simulink model "Speed_State_Feedback_PIL_Simulation"  (R2021b)
settings: Solver=VariableStepAuto  StartTime=0.0  StopTime=20  RelTol=1e-3  EnableMultiTasking=on
libraries: cstblocks x1
settings Model: SILPILSystemUnderTest=refmodels  ExtModeTrigDuration=10  Creator=UTENTE  LastModifiedBy=UTENTE
settings OptimizationCC: EnhancedBackFolding=on  PassReuseOutputArgsAs=Individual arguments  ZeroExternalMemoryAtStartup=off  ZeroInternalMemoryAtStartup=off  MaxStackSize=64  OptimizeBlockOrder=speed  DifferentSizesBufferReuse=on  OptimizationCustomize=off  EfficientTunableParamExpr=on
settings DebuggingCC: ParameterTunabilityLossMsg=error
settings HardwareCC: ProdBitPerPointer=32  ProdBitPerSizeT=32  ProdBitPerPtrDiffT=32  ProdLargestAtomicInteger=Long  ProdLargestAtomicFloat=Double  ProdWordSize=32  ProdLongLongMode=on  ProdHWDeviceType=ARM Compatible->ARM Cortex
settings SFSimCC: MATLABDynamicMemAlloc=off
settings RTWCC: Description=Embedded Coder  SystemTargetFile=ert.tlc  HardwareBoard=STM32 Nucleo F401RE  TemplateMakefile=ert_default_tmf  Toolchain=GNU Tools for ARM Embedded Processors  PortableWordSizes=on  CodeExecutionProfiling=on  CodeProfilingInstrumentation=coarse
settings CodeAppCC: ForceParamTrailComments=on  IgnoreCustomStorageClasses=off  OperatorAnnotations=on  SimulinkDataObjDesc=on  SFDataObjDesc=on  InsertBlockDesc=on
settings ERTTargetCC: ExtModeTransport=3  ExtModeStaticAlloc=on  ExtModeStaticAllocSize=2000  ExtModeMexFile=ext_xcp  ExtModeIntrfLevel=Level2 - Open

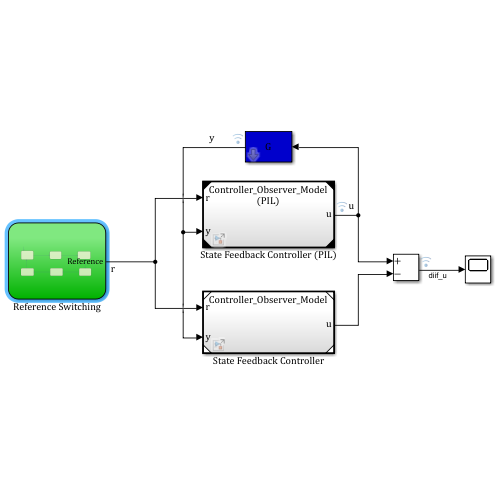
[thumbnail: Simulink's stored preview of the top-level diagram]
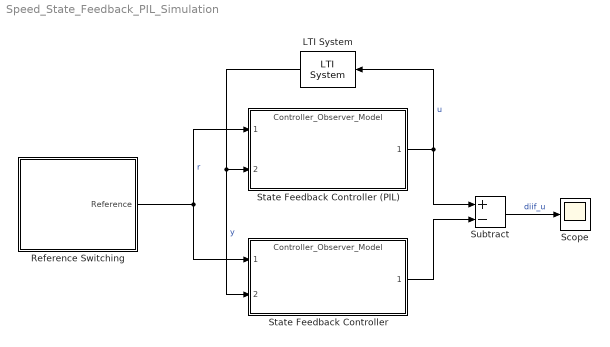
== system Speed_State_Feedback_PIL_Simulation ==
  LTI System : cstblocks/LTI System  sys=G  IC=[]
  Reference Switching : Stateflow chart  TreatAsAtomicUnit=on
  Scope : Scope
  State Feedback Controller : ModelReference  ModelNameDialog=Controller_Observer_Model.slx  SimulationMode=Normal  ModelReferenceVersion=1.6
  State Feedback Controller (PIL) : ModelReference  ModelNameDialog=Controller_Observer_Model.slx  SimulationMode=Processor-in-the-loop (PIL)  ModelReferenceVersion=1.6
  Subtract : Sum  Inputs=+-
  wires:
  Reference Switching/1(Reference) -> State Feedback Controller (PIL)/1, State Feedback Controller/1  "r"
  LTI System/1 -> State Feedback Controller/2, State Feedback Controller (PIL)/2  "y"
  State Feedback Controller/1 -> Subtract/2
  State Feedback Controller (PIL)/1 -> LTI System/1, Subtract/1  "u"
  Subtract/1 -> Scope/1  "diif_u"

== stateflow chart Speed_State_Feedback_PIL_Simulation/Reference Switching ==
  state S1
    Reference=0;
  state S2
    Reference=80;
  state S3
    Reference=125;
  state s7
    Reference=-125;
  state s6
    Reference=-80;
  state s5
    Reference=0;
  (default) -> S1
  S1 -> S2 : after(2,sec)
  S2 -> S3 : after(2,sec)
  S3 -> s5 : after(2,sec)
  s7 -> S1 : after(2,sec)
  s6 -> s7 : after(2,sec)
  s5 -> s6 : after(2,sec)
  data: Reference output
